simulink model "knock0old"  (R2013b)
settings: Solver=FixedStepDiscrete  StartTime=0.0  StopTime=10000  FixedStep=1  RelTol=1e-3
values from neighbouring files (symbols this model uses):
  advanceGain = m1*Delta    (= 0.015)    [plotDriver.m]
  initialSpark = 1.6    [plotDriver.m]
  retardGain = m2*Delta    (= 1.485)    [plotDriver.m]
undefined symbols (not defined in the file): pTarg
settings Model: Creator=jpeytonj  LastModifiedBy=jpeytonj
settings DataIOCC: LimitDataPoints=off  SaveFormat=Structure  SignalLoggingSaveFormat=ModelDataLogs
settings OptimizationCC: InitFltsAndDblsToZero=on
settings DebuggingCC: SaveWithParameterizedLinksMsg=none  SignalResolutionControl=TryResolveAllWithWarning  MultiTaskDSMMsg=warning  MultiTaskCondExecSysMsg=none  FcnCallInpInsideContextMsg=UseLocalSettings
settings SFSimCC: SimParseCustomCode=off
settings RTWCC: IncludeERTFirstTime=on
settings GRTTargetCC: TargetFcnLib=ansi_tfl_tmw.mat  CombineOutputUpdateFcns=off  GRTInterface=on

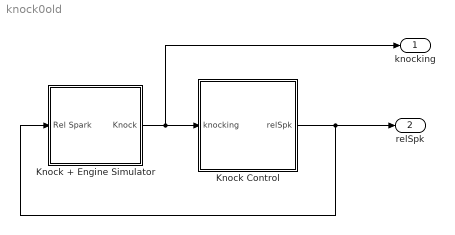
== system knock0old ==
  Knock + Engine Simulator : Subsystem
  Knock Control : Subsystem  TreatAsAtomicUnit=on  mask{initialSpark=initialSpark, retardGain=retardGain, advanceGain=advanceGain, p=pTarg, hiThreshold=2, loThreshold=-2}
      mask prompts: retardGain "Retard Gain:"; advanceGain "Advance Gain:"; p "Desired Knock Probability:"; hiThreshold "CumSum Hi Threshold:"; loThreshold "CumSum Lo Threshold:"
  knocking : Outport
  relSpk : Outport  Port=2
  wires:
  Knock + Engine Simulator/1(Knock) -> Knock Control/1(knocking), knocking/1
  Knock Control/1(relSpk) -> Knock + Engine Simulator/1(Rel Spark), relSpk/1

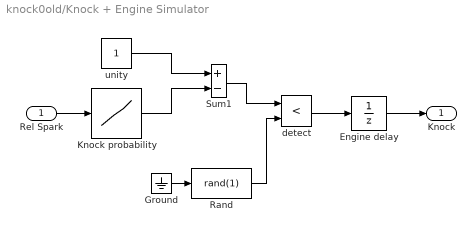
== system knock0old/Knock + Engine Simulator ==
  Rel Spark : Inport
  Engine delay : UnitDelay
  Ground : Ground
  Knock probability : Lookup  InputValues=[-3,-2.9,-2.8,-2.7,-2.6,-2.5,-2.4,-2.3,-2.2,-2.1,-2,-1.9,-1.8,-1.7,-1.6,-1.5,-1.4,-1.3,-1.2,-1.1,-1,-0.9,-0.8,-0.7,-0.6,-0.5,-0.4,-0.3,-0.2,-0.1,0,0.1,0.2,0.3,0.4,0.5,0.6,0.7,0.8,0.9,1,1.1,1.2,1.3,1.4,1.5,1.6,1.7,1.8,1.9,2,2.1,2.2,2.3,2.4,2.5,2.6,2.7,2.8,2.9,3]  Table=[0,0,0,0,0,0,0,0,0,0,0,0.0000118,0.0000463,0.0001024,0.0001788,0.0002745,0.000388,0.0005184,0.0006643,0.0008246,0.001,0.0012,0.0016,0.0021,0.0028,0.0036,0.0046,0.0057,0.007,0.0084,0.01,0.0134,0.0202,0.0297,0.0417,0.0556,0.0711,0.0877,0.1049,0.1224,0.1397,0.1577,0.1776,0.1992,0.2224,0.2471,0.2732,0.3006,0.3291,0.3587,0.3892,0.4206,0.4526,0.4852,0.5183,0.5518,0.5855,0.6194,0.6533,0.6871,0.7207]
  Rand : MATLABFcn  MATLABFcn=rand(1)  OutputDimensions=1  SampleTime=[1 0]
  Sum1 : Sum  Inputs=+-
  detect : RelationalOperator  Operator=<  OutDataTypeStr=boolean
  unity : Constant
  Knock : Outport
  wires:
  unity/1 -> Sum1/1
  Knock probability/1 -> Sum1/2
  Sum1/1 -> detect/1
  Rel Spark/1 -> Knock probability/1
  detect/1 -> Engine delay/1
  Engine delay/1 -> Knock/1
  Rand/1 -> detect/2
  Ground/1 -> Rand/1

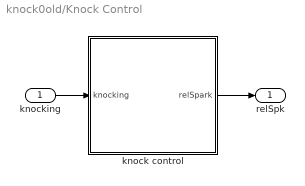
== system knock0old/Knock Control ==
  knocking : Inport
  knock control : MATLAB Function  TreatAsAtomicUnit=on
  relSpk : Outport
  wires:
  knock control/1(relSpark) -> relSpk/1
  knocking/1 -> knock control/1(knocking)

== matlab function knock0old/Knock Control/knock control ==
  data: knocking input; initialSpark parameter; relSpark output; retardGain parameter; advanceGain parameter
function relSpark = knCtrl(knocking,initialSpark,retardGain,advanceGain)

%Computes the new relative spark angle (deg) based on:
%   knocking:       a boolean knock signal
%   initialSpark:   the initial spark relative to borderline
%   retardGain:     the retard amount (deg)
%   advanceGain     the advance amount (deg)

%   Copyright 2009 Villanova University
%   Author: James C. Peyton Jones  (5/1/2009)
%   Version knock0:  Traditional Knock Control
%   Revision:        Date:
%
%

%Declare persistent variables
persistent relSpk

%Initialization
if isempty(relSpk),
    relSpk= double(initialSpark);
end;

%Traditional knock control
if knocking,
	relSpk= relSpk - retardGain;
else
	relSpk= relSpk + advanceGain;
end;

%Apply saturation limits
if relSpk>4, relSpk=4; end;
if relSpk<-4, relSpk=-4; end;

%Output value
relSpark= double(relSpk);
